simulink model "SP_DC_Model"  (R2014a)
settings: Solver=ode15s  StartTime=0.0  StopTime=10  MaxStep=1  RelTol=1e-9
values from neighbouring files (symbols this model uses):
  DC_M =     [matlab.mat]
libraries: fl_lib x7, nesl_utility x5, elec_lib x1
settings Model: Creator=Staszko  LastModifiedBy=Staszko

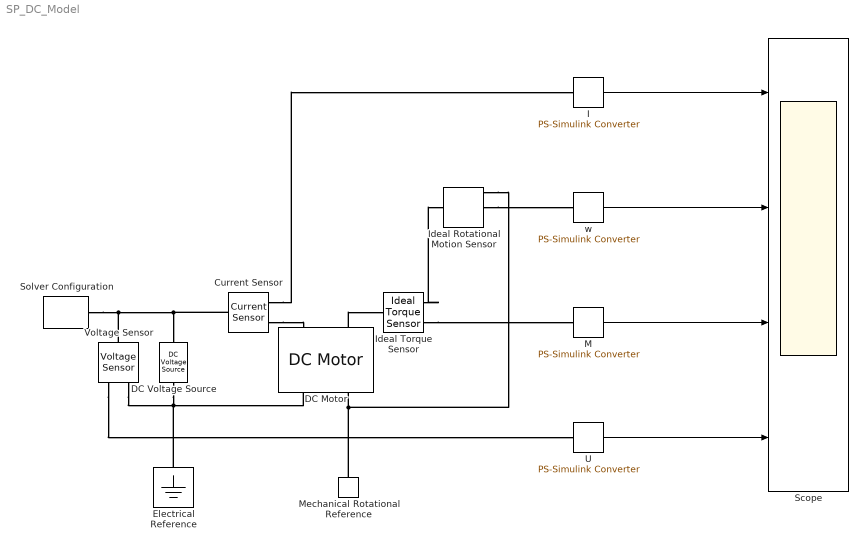
== system SP_DC_Model ==
  Current Sensor : fl_lib/Electrical/Electrical Sensors/Current Sensor
  DC Motor : elec_lib/Actuators & Drivers/Rotational Actuators/DC Motor  parameterization=1  Ra=DC_M.Rt Ohm  La=DC_M.Lt H  emf_or_torque=2  Kv=7.2e-5 V/rpm  Ki=DC_M.M_const N*m/A  T_stall=2.4e-4 N*m  w_max=1.91e+4 rpm  w_rated=1.5e+4 rpm  P_rated=0.08 W  V_rated=1.5 V  J=DC_M.J kg*m^2  lam_param=2  lam=5 N*m/(rad/s)  i_noload=DC_M.I_iddle A  V_i_noload=DC_M.Un V  speed0=0 rpm  alpha=0.00393 1/K  Tmeas=25 C  thermal_mass=100 J/K  initial_temperature=25 C
  DC Voltage Source : fl_lib/Electrical/Electrical Sources/DC Voltage Source  v0=DC_M.Un V
  Electrical Reference : fl_lib/Electrical/Electrical Elements/Electrical Reference
  I : nesl_utility/PS-Simulink Converter  PhysicalDomain=network_engine_domain  SubClassName=ps_output  LeftPortType=input  RightPortType=output  PseudoPeriodic=off  Frequencies=[]  Unit=1  AffineConversion=off
  Ideal Rotational Motion Sensor : fl_lib/Mechanical/Mechanical Sensors/Ideal Rotational Motion Sensor  offset=0 rad
  Ideal Torque Sensor : fl_lib/Mechanical/Mechanical Sensors/Ideal Torque Sensor
  M : nesl_utility/PS-Simulink Converter  PhysicalDomain=network_engine_domain  SubClassName=ps_output  LeftPortType=input  RightPortType=output  PseudoPeriodic=off  Frequencies=[]  Unit=1  AffineConversion=off
  Mechanical Rotational Reference : fl_lib/Mechanical/Rotational Elements/Mechanical Rotational Reference
  Scope : Scope  NumInputPorts=4
      settings: ShowLegends=on  YMin=-5~-5~-5~-5  YMax=5~5~5~5
  Solver Configuration : nesl_utility/Solver Configuration  PhysicalDomain=network_engine_domain  SubClassName=solver  LeftPortType=input  RightPortType=generic  Accelerate=off  Tones=[]  Harmonics=[]  SimulateNoise=off  Profile=off  UseLocalSampling=off  EnableSwitchedLinearOptims=on  FrequencyDomain=off  UseCCode=off  RelTol=0.001  AbsTol=1e-06  MinStep=1e-09  ToWorkspace=off  DoDC=off  ResidualTolerance=1e-09  UseLocalSolver=off  LocalSolverChoice=NE_BACKWARD_EULER_ADVANCER  LocalSolverSampleTime=0.001  DoFixedCost=off  MaxNonlinIter=3  MaxModeIter=2  LinearAlgebra=Sparse  DelaysMemoryBudget=1024  AutomaticFiltering=on  FilteringTimeConstant=0.001
  U : nesl_utility/PS-Simulink Converter  PhysicalDomain=network_engine_domain  SubClassName=ps_output  LeftPortType=input  RightPortType=output  PseudoPeriodic=off  Frequencies=[]  Unit=1  AffineConversion=off
  Voltage Sensor : fl_lib/Electrical/Electrical Sensors/Voltage Sensor
  w : nesl_utility/PS-Simulink Converter  PhysicalDomain=network_engine_domain  SubClassName=ps_output  LeftPortType=input  RightPortType=output  PseudoPeriodic=off  Frequencies=[]  Unit=1  AffineConversion=off
  wires:
  I/1 -> Scope/1
  w/1 -> Scope/2
  M/1 -> Scope/3
  U/1 -> Scope/4
  connections:
  Solver Configuration/RConn1 -- Voltage Sensor/LConn1 -- Current Sensor/LConn1 -- DC Voltage Source/LConn1
  DC Voltage Source/RConn1 -- Electrical Reference/LConn1 -- DC Motor/RConn1 -- Voltage Sensor/RConn2
  Ideal Rotational Motion Sensor/RConn1 -- Mechanical Rotational Reference/LConn1 -- DC Motor/RConn2
  Current Sensor/RConn2 -- DC Motor/LConn1
  Current Sensor/RConn1 -- I/LConn1
  Voltage Sensor/RConn1 -- U/LConn1
  Ideal Rotational Motion Sensor/RConn2 -- w/LConn1
  Ideal Torque Sensor/RConn2 -- M/LConn1
  DC Motor/LConn2 -- Ideal Torque Sensor/LConn1
  Ideal Torque Sensor/RConn1 -- Ideal Rotational Motion Sensor/LConn1
